simulink model "simulink_discrete_3_R2021a"  (R2021a)
settings: Solver=ode45  StartTime=0.0  StopTime=0.7  RelTol=1e-3  EnableMultiTasking=on
libraries: cstblocks x6, simulink x2, dsparch4 x1
settings Model: Creator=Koldo  LastModifiedBy=Koldo
settings SolverCC: AlgebraicLoopSolver=TrustRegion
settings DataIOCC: LimitDataPoints=on  SaveFormat=Array  SignalLoggingSaveFormat=ModelDataLogs  ReturnWorkspaceOutputs=off
settings OptimizationCC: ExpressionDepthLimit=2147483647  LifeSpan=inf
settings DebuggingCC: UnderspecifiedInitializationDetection=Classic  MergeDetectMultiDrivingBlocksExec=none  SolverPrmCheckMsg=warning  FcnCallInpInsideContextMsg=warning  StateNameClashWarn=warning  SFUnexpectedBacktrackingDiag=warning  SFNoUnconditionalDefaultTransitionDiag=warning  SFExecutionAtInitializationDiag=none  SFMachineParentedDataDiag=warning  ArithmeticOperatorsInVariantConditions=warning
settings HardwareCC: ProdBitPerPointer=32  ProdBitPerSizeT=32  ProdBitPerPtrDiffT=32  ProdLargestAtomicFloat=None  ProdIntDivRoundTo=Undefined  ProdEndianess=Unspecified  ProdWordSize=32  ProdHWDeviceType=32-bit Generic
settings ModelReferenceCC: PropagateSignalLabelsOutOfModel=off
settings SFSimCC: SimUseLocalCustomCode=off  CustomCodeUndefinedFunction=UseInterfaceOnly
settings RTWCC: RTWUseLocalCustomCode=off
settings CodeAppCC: StateflowObjectComments=on
settings GRTTargetCC: TargetLangStandard=C89/C90 (ANSI)  CombineOutputUpdateFcns=off  GRTInterface=on
settings ConfigComp: CovMetricSettings=dw  CovSaveCumulativeToWorkspaceVar=on  CovSaveSingleToWorkspaceVar=on  CovExternalEMLEnable=off

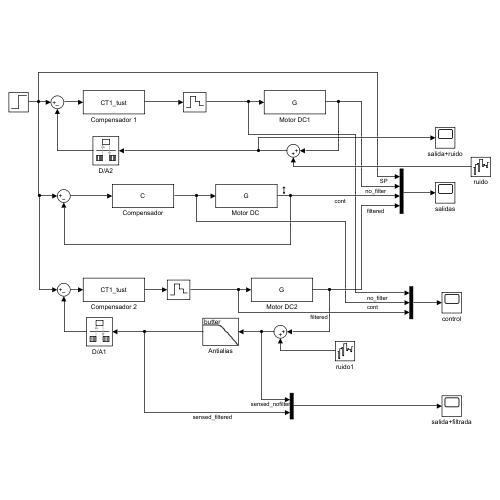
[thumbnail: Simulink's stored preview of the top-level diagram]
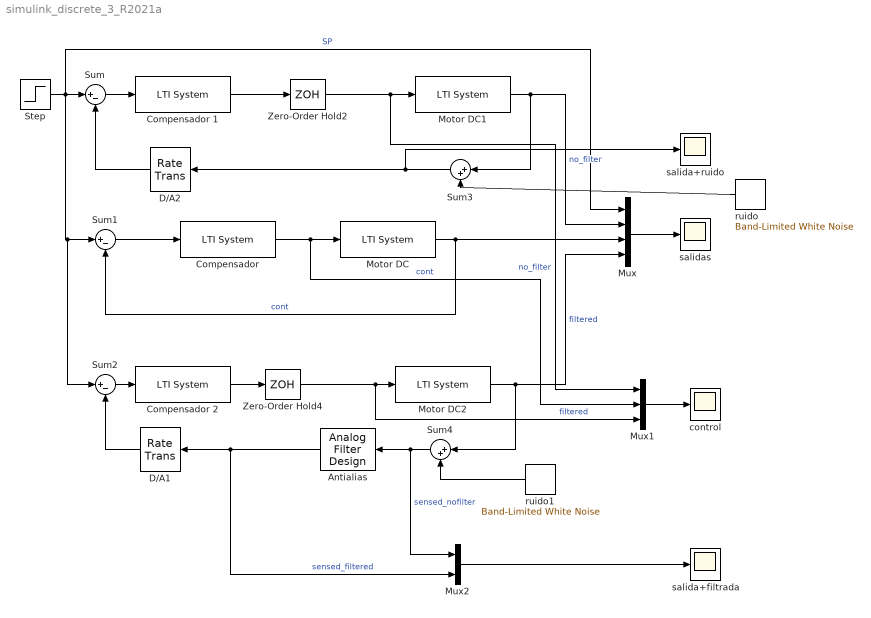
== system simulink_discrete_3_R2021a ==
  Antialias : dsparch4/Analog Filter Design  method=Butterworth  filttype=Lowpass  N=4  Wlo=100  Whi=80  Rp=2  Rs=40
  Compensador : cstblocks/LTI System  sys=C  IC=[]
  Compensador 1 : cstblocks/LTI System  sys=CT1_tust  IC=[]
  Compensador 2 : cstblocks/LTI System  sys=CT1_tust  IC=[]
  D/A1 : RateTransition  Integrity=off  Deterministic=off  InitialCondition=8.96  OutPortSampleTime=T1
  D/A2 : RateTransition  Integrity=off  Deterministic=off  InitialCondition=8.96  OutPortSampleTime=T1
  "Motor DC " : cstblocks/LTI System  sys=G  IC=[]
  Motor DC1 : cstblocks/LTI System  sys=G  IC=[]
  Motor DC2 : cstblocks/LTI System  sys=G  IC=[]
  Mux : Mux
  Mux1 : Mux  Inputs=3
  Mux2 : Mux  Inputs=2
  Step : Step  Time=0.1  After=pi/2  SampleTime=0
  Sum : Sum  Inputs=|+-
  Sum1 : Sum  Inputs=|+-
  Sum2 : Sum  Inputs=|+-
  Sum3 : Sum  Inputs=|++
  Sum4 : Sum  Inputs=|++
  Zero-Order Hold2 : ZeroOrderHold  SampleTime=-1
  Zero-Order Hold4 : ZeroOrderHold  SampleTime=-1
  control : Scope
  ruido : simulink/Sources/Band-Limited White Noise  Cov=[0.0000001]  Ts=0.0001  seed=[23341]
  ruido1 : simulink/Sources/Band-Limited White Noise  Cov=[0.0000001]  Ts=0.0001  seed=[23341]
  salida+filtrada : Scope
  salida+ruido : Scope
  salidas : Scope
  wires:
  Sum/1 -> Compensador 1/1
  Motor DC1/1 -> Mux/2, Sum3/1  "no_filter"
  Compensador 1/1 -> Zero-Order Hold2/1
  Zero-Order Hold2/1 -> Motor DC1/1, Mux1/1  "no_filter"
  Sum1/1 -> Compensador/1
  "Motor DC "/1 -> Mux/3, Sum1/2  "cont"
  Compensador/1 -> "Motor DC "/1, Mux1/2  "cont"
  Mux/1 -> salidas/1
  Step/1 -> Sum2/1, Sum1/1, Mux/1, Sum/1  "SP"
  Sum2/1 -> Compensador 2/1
  Motor DC2/1 -> Mux/4, Sum4/1  "filtered"
  Zero-Order Hold4/1 -> Motor DC2/1, Mux1/3  "filtered"
  Mux1/1 -> control/1
  D/A1/1 -> Sum2/2
  Compensador 2/1 -> Zero-Order Hold4/1
  Sum3/1 -> salida+ruido/1, D/A2/1
  ruido/1 -> Sum3/2
  Sum4/1 -> Antialias/1, Mux2/1  "sensed_nofilter"
  Antialias/1 -> Mux2/2, D/A1/1  "sensed_filtered"
  ruido1/1 -> Sum4/2
  Mux2/1 -> salida+filtrada/1
  D/A2/1 -> Sum/2
